simulink model "problem4filter"  (R2020b)
settings: Solver=VariableStepAuto  StartTime=0.0  StopTime=10.0  RelTol=1e-3
settings Model: Creator=Shivashis  LastModifiedBy=Shivashis

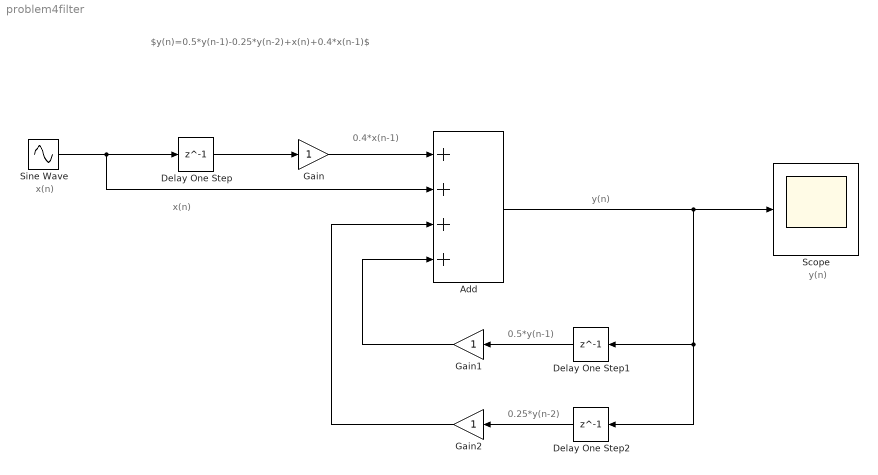
== system problem4filter ==
  note: y(n)
  note: x(n)
  note: $y(n)=0.5*y(n-1)-0.25*y(n-2)+x(n)+0.4*x(n-1)$
  note: x(n)
  note: 0.4*x(n-1)
  note: 0.5*y(n-1)
  note: 0.25*y(n-2)
  note: y(n)
  Add : Sum  Inputs=++++
  Delay One Step : Delay  DelayLength=1
  Delay One Step1 : Delay  DelayLength=1
  Delay One Step2 : Delay  DelayLength=1
  Gain : Gain
  Gain1 : Gain
  Gain2 : Gain
  Scope : Scope
  Sine Wave : Sin  SampleTime=0
  wires:
  Sine Wave/1 -> Add/2, Delay One Step/1
  Delay One Step/1 -> Gain/1
  Gain/1 -> Add/1
  Add/1 -> Delay One Step2/1, Delay One Step1/1, Scope/1
  Delay One Step1/1 -> Gain1/1
  Delay One Step2/1 -> Gain2/1
  Gain2/1 -> Add/3
  Gain1/1 -> Add/4
